simulink model "test"  (R2016a)
settings: Solver=VariableStepAuto  StartTime=0.0  StopTime=1  MaxStep=0.001  RelTol=1e-3
values from neighbouring files (symbols this model uses):
  A = 40    [Courbe2d.m]    (also in Donneesp2.m; main.m)
  Ceq = 2*zeta*sqrt(Keq*Meq)    [main.m]
  I = 25    [main.m]
  Keq = k*(d^2)    (= 400000)    [main.m]
  v0 = 0    [Donneesp2.m]    (also in main.m)
  w = 50    [Donneesp2.m]    (also in main.m = Wn)
  x0 = 0    [Donneesp2.m]    (also in main.m)
settings Model: Creator=mohacg  LastModifiedBy=mohacg

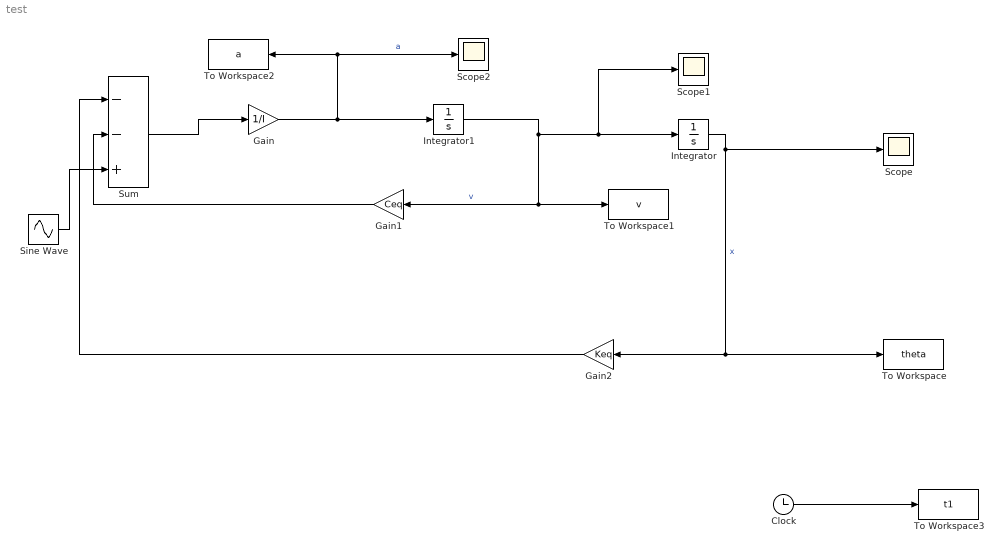
== system test ==
  Clock : Clock
  Gain : Gain  Gain=1/I
  Gain1 : Gain  Gain=Ceq
  Gain2 : Gain  Gain=Keq
  Integrator : Integrator  InitialCondition=x0
  Integrator1 : Integrator  InitialCondition=v0
  Scope : Scope
  Scope1 : Scope
  Scope2 : Scope
  Sine Wave : Sin  Amplitude=A  Frequency=w  SampleTime=0
  Sum : Sum  Inputs=|--+
  To Workspace : ToWorkspace  VariableName=theta  SampleTime=-1
  To Workspace1 : ToWorkspace  VariableName=v  SampleTime=-1
  To Workspace2 : ToWorkspace  VariableName=a  SampleTime=-1
  To Workspace3 : ToWorkspace  VariableName=t1  SampleTime=-1
  wires:
  Gain/1 -> To Workspace2/1, Scope2/1, Integrator1/1  "a"
  Integrator1/1 -> To Workspace1/1, Gain1/1, Scope1/1, Integrator/1  "v"
  Integrator/1 -> To Workspace/1, Gain2/1, Scope/1  "x"
  Sum/1 -> Gain/1
  Gain1/1 -> Sum/2
  Gain2/1 -> Sum/1
  Clock/1 -> To Workspace3/1
  Sine Wave/1 -> Sum/3
